simulink model "QuadrotorSimulink"  (Simulink 9.0)
settings: Solver=ode45  StartTime=0.0  StopTime=10  RelTol=1e-3  EnableMultiTasking=on
undefined symbols (not defined in the file): Quad
settings Model: Creator=test  LastModifiedBy=Dariush
settings DataIOCC: LimitDataPoints=on  SignalLoggingSaveFormat=ModelDataLogs
settings OptimizationCC: ExpressionDepthLimit=2147483647
settings DebuggingCC: FcnCallInpInsideContextMsg=warning  StateNameClashWarn=warning  StrictBusMsg=Warning
settings GRTTargetCC: CombineOutputUpdateFcns=off  GRTInterface=on

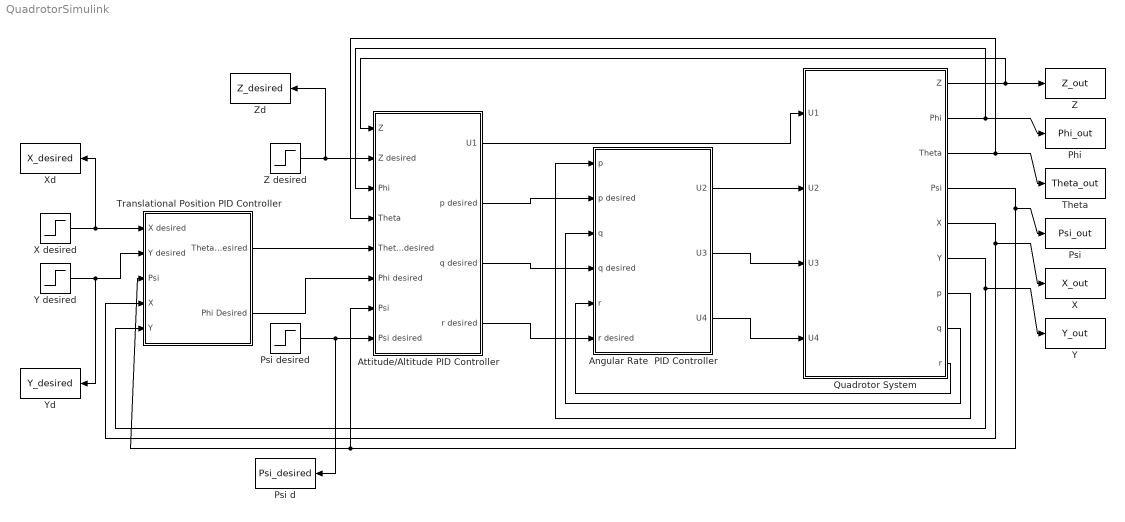
== system QuadrotorSimulink ==
  Angular Rate  PID Controller : Subsystem
  Attitude/Altitude PID Controller : Subsystem
  Phi : ToWorkspace  VariableName=Phi_out  SaveFormat=Structure  SampleTime=-1
  Psi : ToWorkspace  VariableName=Psi_out  SaveFormat=Structure  SampleTime=-1
  Psi d : ToWorkspace  VariableName=Psi_desired  SaveFormat=Structure  SampleTime=-1
  Psi desired : Step  After=0  SampleTime=0
  Quadrotor System : Subsystem
  Theta : ToWorkspace  VariableName=Theta_out  SaveFormat=Structure  SampleTime=-1
  Translational Position PID Controller : Subsystem
  X : ToWorkspace  VariableName=X_out  SaveFormat=Structure  SampleTime=-1
  X desired : Step  After=.25  SampleTime=0
  Xd : ToWorkspace  VariableName=X_desired  SaveFormat=Structure  SampleTime=-1
  Y : ToWorkspace  VariableName=Y_out  SaveFormat=Structure  SampleTime=-1
  Y desired : Step  After=0  SampleTime=0
  Yd : ToWorkspace  VariableName=Y_desired  SaveFormat=Structure  SampleTime=-1
  Z : ToWorkspace  VariableName=Z_out  SaveFormat=Structure  SampleTime=-1
  Z desired : Step  After=.5  SampleTime=0
  Zd : ToWorkspace  VariableName=Z_desired  SaveFormat=Structure  SampleTime=-1
  wires:
  Quadrotor System/2(Phi) -> Phi/1, Attitude/Altitude PID Controller/3(Phi)
  Quadrotor System/3(Theta) -> Attitude/Altitude PID Controller/4(Theta), Theta/1
  Quadrotor System/4(Psi) -> Psi/1, Translational Position PID Controller/3(Psi), Attitude/Altitude PID Controller/7(Psi)
  Quadrotor System/5(X) -> X/1, Translational Position PID Controller/4(X)
  Quadrotor System/6(Y) -> Y/1, Translational Position PID Controller/5(Y)
  Quadrotor System/1(Z) -> Attitude/Altitude PID Controller/1(Z), Z/1
  Psi desired/1 -> Attitude/Altitude PID Controller/8(Psi desired), Psi d/1
  Z desired/1 -> Attitude/Altitude PID Controller/2(Z desired), Zd/1
  X desired/1 -> Translational Position PID Controller/1(X desired), Xd/1
  Y desired/1 -> Yd/1, Translational Position PID Controller/2(Y desired)
  Attitude/Altitude PID Controller/1(U1) -> Quadrotor System/1(U1)
  Translational Position PID Controller/1(Theta Desired) -> Attitude/Altitude PID Controller/5(Theta desired)
  Translational Position PID Controller/2(Phi Desired) -> Attitude/Altitude PID Controller/6(Phi desired)
  Attitude/Altitude PID Controller/2(p desired) -> Angular Rate  PID Controller/2(p desired)
  Attitude/Altitude PID Controller/3(q desired) -> Angular Rate  PID Controller/4(q desired)
  Attitude/Altitude PID Controller/4(r desired) -> Angular Rate  PID Controller/6(r desired)
  Quadrotor System/9(r) -> Angular Rate  PID Controller/5(r)
  Quadrotor System/8(q) -> Angular Rate  PID Controller/3(q)
  Quadrotor System/7(p) -> Angular Rate  PID Controller/1(p)
  Angular Rate  PID Controller/3(U4) -> Quadrotor System/4(U4)
  Angular Rate  PID Controller/2(U3) -> Quadrotor System/3(U3)
  Angular Rate  PID Controller/1(U2) -> Quadrotor System/2(U2)

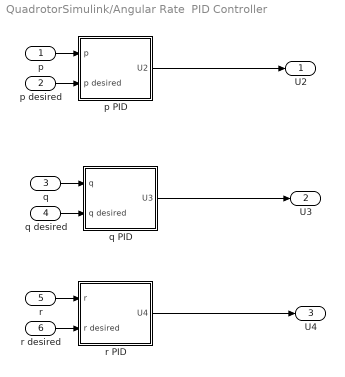
== system QuadrotorSimulink/Angular Rate  PID Controller ==
  p : Inport
  p desired : Inport  Port=2
  q : Inport  Port=3
  q desired : Inport  Port=4
  r : Inport  Port=5
  r desired : Inport  Port=6
  p PID : Subsystem
  q PID : Subsystem
  r PID : Subsystem
  U2 : Outport
  U3 : Outport  Port=2
  U4 : Outport  Port=3
  wires:
  p PID/1(U2) -> U2/1
  q PID/1(U3) -> U3/1
  r PID/1(U4) -> U4/1
  p/1 -> p PID/1(p)
  p desired/1 -> p PID/2(p desired)
  q/1 -> q PID/1(q)
  q desired/1 -> q PID/2(q desired)
  r/1 -> r PID/1(r)
  r desired/1 -> r PID/2(r desired)

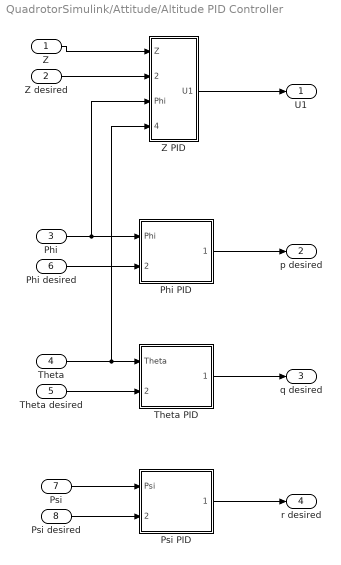
== system QuadrotorSimulink/Attitude/Altitude PID Controller ==
  Z : Inport
  Z desired : Inport  Port=2
  Phi : Inport  Port=3
  Theta : Inport  Port=4
  Theta desired : Inport  Port=5
  Phi desired : Inport  Port=6
  Psi : Inport  Port=7
  Psi desired : Inport  Port=8
  Phi PID : Subsystem
  Psi PID : Subsystem
  Theta PID : Subsystem
  Z PID : Subsystem
  U1 : Outport
  p desired : Outport  Port=2
  q desired : Outport  Port=3
  r desired : Outport  Port=4
  wires:
  Z PID/1(U1) -> U1/1
  Z desired/1 -> Z PID/2(Z desired)
  Z/1 -> Z PID/1(Z)
  Phi desired/1 -> Phi PID/2(Phi desired)
  Phi/1 -> Phi PID/1(Phi), Z PID/3(Phi)
  Psi desired/1 -> Psi PID/2(Psi desired)
  Psi/1 -> Psi PID/1(Psi)
  Theta desired/1 -> Theta PID/2(Theta desired)
  Theta/1 -> Theta PID/1(Theta), Z PID/4(Theta)
  Phi PID/1(p desired) -> p desired/1
  Psi PID/1(r desired) -> r desired/1
  Theta PID/1(q desired) -> q desired/1

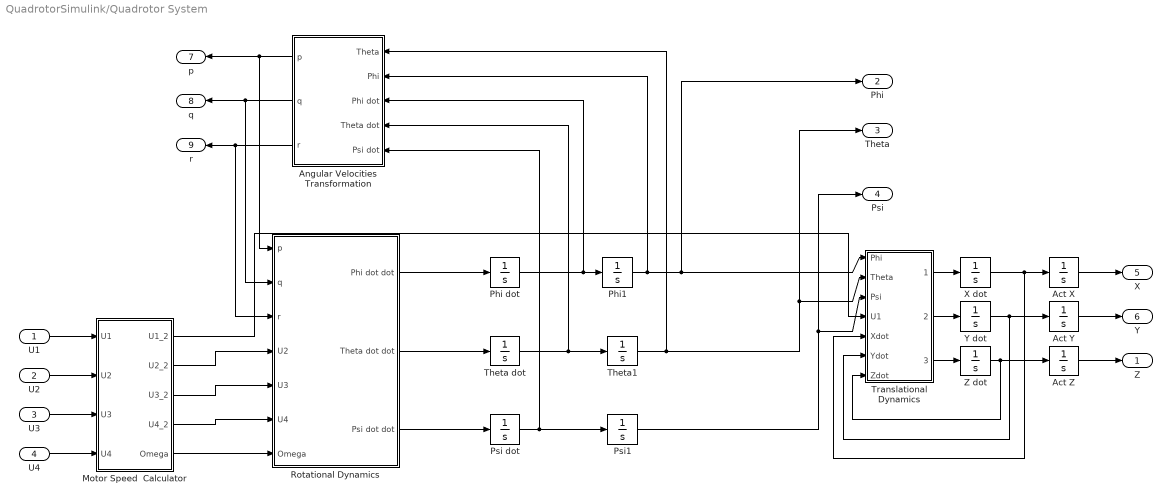
== system QuadrotorSimulink/Quadrotor System ==
  U1 : Inport
  U2 : Inport  Port=2
  U3 : Inport  Port=3
  U4 : Inport  Port=4
  Act X : Integrator
  Act Y : Integrator
  Act Z : Integrator
  Angular Velocities Transformation : Subsystem
  Motor Speed  Calculator : Subsystem
  Phi dot : Integrator
  Phi1 : Integrator  ZeroCross=off
  Psi dot : Integrator  ZeroCross=off
  Psi1 : Integrator  ZeroCross=off
  Rotational Dynamics : Subsystem
  Theta dot : Integrator  ZeroCross=off
  Theta1 : Integrator  ZeroCross=off
  Translational Dynamics : Subsystem
  X dot : Integrator
  Y dot : Integrator
  Z dot : Integrator
  Z : Outport
  Phi : Outport  Port=2
  Theta : Outport  Port=3
  Psi : Outport  Port=4
  X : Outport  Port=5
  Y : Outport  Port=6
  p : Outport  Port=7
  q : Outport  Port=8
  r : Outport  Port=9
  wires:
  Rotational Dynamics/2(Theta dot dot) -> Theta dot/1
  Motor Speed  Calculator/5(Omega) -> Rotational Dynamics/7(Omega)
  Phi1/1 -> Translational Dynamics/1(Phi), Phi/1, Angular Velocities Transformation/2(Phi)
  Theta1/1 -> Translational Dynamics/2(Theta), Theta/1, Angular Velocities Transformation/1(Theta)
  Psi1/1 -> Translational Dynamics/3(Psi), Psi/1
  Translational Dynamics/1(x dotdot) -> X dot/1
  X dot/1 -> Act X/1, Translational Dynamics/5(Xdot)
  Y dot/1 -> Act Y/1, Translational Dynamics/6(Ydot)
  Translational Dynamics/2(y dotdot) -> Y dot/1
  Z dot/1 -> Translational Dynamics/7(Zdot), Act Z/1
  Translational Dynamics/3(z dotdot) -> Z dot/1
  Act X/1 -> X/1
  Act Y/1 -> Y/1
  Act Z/1 -> Z/1
  Psi dot/1 -> Psi1/1, Angular Velocities Transformation/5(Psi dot)
  Theta dot/1 -> Theta1/1, Angular Velocities Transformation/4(Theta dot)
  Phi dot/1 -> Phi1/1, Angular Velocities Transformation/3(Phi dot)
  Rotational Dynamics/3(Psi dot dot) -> Psi dot/1
  Rotational Dynamics/1(Phi dot dot) -> Phi dot/1
  U4/1 -> Motor Speed  Calculator/4(U4)
  U2/1 -> Motor Speed  Calculator/2(U2)
  U3/1 -> Motor Speed  Calculator/3(U3)
  Motor Speed  Calculator/2(U2_2) -> Rotational Dynamics/4(U2)
  Motor Speed  Calculator/3(U3_2) -> Rotational Dynamics/5(U3)
  Motor Speed  Calculator/1(U1_2) -> Translational Dynamics/4(U1)
  Motor Speed  Calculator/4(U4_2) -> Rotational Dynamics/6(U4)
  Angular Velocities Transformation/1(p) -> Rotational Dynamics/1(p), p/1
  Angular Velocities Transformation/2(q) -> Rotational Dynamics/2(q), q/1
  Angular Velocities Transformation/3(r) -> Rotational Dynamics/3(r), r/1
  U1/1 -> Motor Speed  Calculator/1(U1)

== system QuadrotorSimulink/Translational Position PID Controller ==
  X desired : Inport
  Y desired : Inport  Port=2
  Psi : Inport  Port=3
  X : Inport  Port=4
  Y : Inport  Port=5
  Desired Position GF to BF : Subsystem
  Position GF to BF : Subsystem
  X PID : Subsystem
  Y PID : Subsystem
  Theta Desired : Outport
  Phi Desired : Outport  Port=2
  wires:
  X PID/1(Theta Desired) -> Theta Desired/1
  Y PID/1(Phi Desired) -> Phi Desired/1
  X desired/1 -> Desired Position GF to BF/1(X GF)
  Y desired/1 -> Desired Position GF to BF/2(Y GF)
  Desired Position GF to BF/1("X Bf ") -> X PID/1(X desired)
  Desired Position GF to BF/2(Y Bf) -> Y PID/1(Y desired)
  X/1 -> Position GF to BF/1(X GF)
  Y/1 -> Position GF to BF/2(Y GF)
  Position GF to BF/1("X Bf ") -> X PID/2(X)
  Position GF to BF/2(Y Bf) -> Y PID/2(Y)
  Psi/1 -> Desired Position GF to BF/3(Psi), Position GF to BF/3(Psi)

== system QuadrotorSimulink/Angular Rate  PID Controller/p PID ==
  p : Inport
  p desired : Inport  Port=2
  Derivative : Derivative
  Integrator : Integrator
  Kd : Gain  Gain=Quad.p_KD
  Ki : Gain  Gain=Quad.p_KI
  Kp : Gain  Gain=Quad.p_KP
  Psi Error : Sum  Inputs=+-
  Saturation1 : Saturate  UpperLimit=Quad.U2_max  LowerLimit=Quad.U2_min
  Sum : Sum  Inputs=+++
  U2 : Outport
  wires:
  p/1 -> Psi Error/2, Derivative/1
  p desired/1 -> Psi Error/1
  Derivative/1 -> Kd/1
  Kp/1 -> Sum/1
  Sum/1 -> U2/1
  Psi Error/1 -> Integrator/1, Kp/1
  Integrator/1 -> Ki/1
  Kd/1 -> Sum/3
  Ki/1 -> Saturation1/1
  Saturation1/1 -> Sum/2

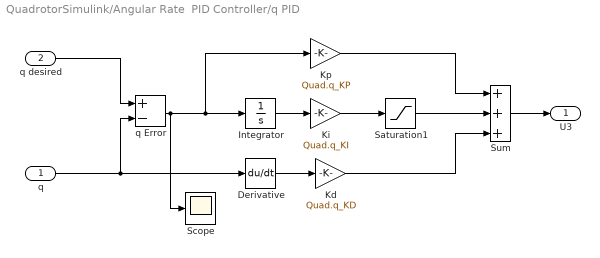
== system QuadrotorSimulink/Angular Rate  PID Controller/q PID ==
  q : Inport
  q desired : Inport  Port=2
  Derivative : Derivative
  Integrator : Integrator
  Kd : Gain  Gain=Quad.q_KD
  Ki : Gain  Gain=Quad.q_KI
  Kp : Gain  Gain=Quad.q_KP
  Saturation1 : Saturate  UpperLimit=Quad.U3_max  LowerLimit=Quad.U3_min
  Scope : Scope
  Sum : Sum  Inputs=+++
  q Error : Sum  Inputs=+-
  U3 : Outport
  wires:
  q/1 -> q Error/2, Derivative/1
  q desired/1 -> q Error/1
  Derivative/1 -> Kd/1
  Kp/1 -> Sum/1
  Sum/1 -> U3/1
  q Error/1 -> Integrator/1, Kp/1, Scope/1
  Integrator/1 -> Ki/1
  Kd/1 -> Sum/3
  Ki/1 -> Saturation1/1
  Saturation1/1 -> Sum/2

== system QuadrotorSimulink/Angular Rate  PID Controller/r PID ==
  r : Inport
  r desired : Inport  Port=2
  Derivative : Derivative
  Integrator : Integrator
  Kd : Gain  Gain=Quad.r_KD
  Ki : Gain  Gain=Quad.r_KI
  Kp : Gain  Gain=Quad.r_KP
  Psi Error : Sum  Inputs=+-
  Sum : Sum  Inputs=+++
  U4 : Outport
  wires:
  r/1 -> Psi Error/2, Derivative/1
  r desired/1 -> Psi Error/1
  Derivative/1 -> Kd/1
  Kp/1 -> Sum/1
  Sum/1 -> U4/1
  Psi Error/1 -> Integrator/1, Kp/1
  Integrator/1 -> Ki/1
  Kd/1 -> Sum/3
  Ki/1 -> Sum/2

== system QuadrotorSimulink/Attitude/Altitude PID Controller/Phi PID ==
  Phi : Inport
  Phi desired : Inport  Port=2
  Derivative : Derivative
  Integrator : Integrator
  Kd : Gain  Gain=Quad.phi_KD
  Ki : Gain  Gain=Quad.phi_KI
  Kp : Gain  Gain=Quad.phi_KP
  Psi Error : Sum  Inputs=+-
  Sum : Sum  Inputs=+++
  p desired : Outport
  wires:
  Phi/1 -> Psi Error/2, Derivative/1
  Phi desired/1 -> Psi Error/1
  Derivative/1 -> Kd/1
  Kp/1 -> Sum/1
  Sum/1 -> p desired/1
  Psi Error/1 -> Integrator/1, Kp/1
  Integrator/1 -> Ki/1
  Kd/1 -> Sum/3
  Ki/1 -> Sum/2

== system QuadrotorSimulink/Attitude/Altitude PID Controller/Psi PID ==
  Psi : Inport
  Psi desired : Inport  Port=2
  Derivative : Derivative
  Integrator : Integrator
  Kd : Gain  Gain=Quad.psi_KD
  Ki : Gain  Gain=Quad.psi_KI
  Kp : Gain  Gain=Quad.psi_KP
  Psi Error : Sum  Inputs=+-
  Sum : Sum  Inputs=+++
  r desired : Outport
  wires:
  Psi/1 -> Psi Error/2, Derivative/1
  Psi desired/1 -> Psi Error/1
  Derivative/1 -> Kd/1
  Kp/1 -> Sum/1
  Sum/1 -> r desired/1
  Psi Error/1 -> Integrator/1, Kp/1
  Integrator/1 -> Ki/1
  Kd/1 -> Sum/3
  Ki/1 -> Sum/2

== system QuadrotorSimulink/Attitude/Altitude PID Controller/Theta PID ==
  Theta : Inport
  Theta desired : Inport  Port=2
  Derivative : Derivative
  Integrator : Integrator
  Kd : Gain  Gain=Quad.theta_KD
  Ki : Gain  Gain=Quad.theta_KI
  Kp : Gain  Gain=Quad.theta_KP
  Scope : Scope
  Sum : Sum  Inputs=+++
  Theta Error : Sum  Inputs=+-
  q desired : Outport
  wires:
  Theta/1 -> Theta Error/2, Derivative/1
  Theta desired/1 -> Theta Error/1
  Derivative/1 -> Kd/1
  Kp/1 -> Sum/1
  Sum/1 -> q desired/1
  Theta Error/1 -> Integrator/1, Kp/1, Scope/1
  Integrator/1 -> Ki/1
  Kd/1 -> Sum/3
  Ki/1 -> Sum/2

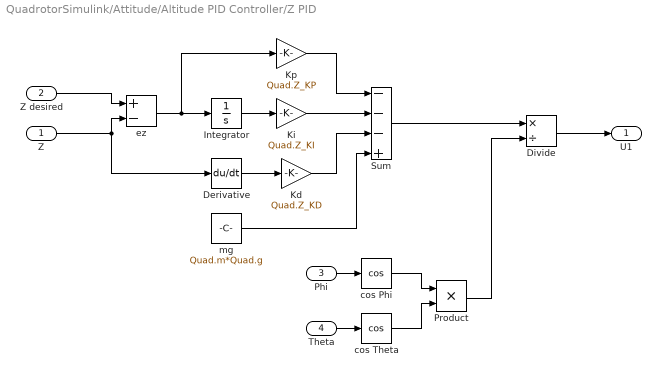
== system QuadrotorSimulink/Attitude/Altitude PID Controller/Z PID ==
  Z : Inport
  Z desired : Inport  Port=2
  Phi : Inport  Port=3
  Theta : Inport  Port=4
  Derivative : Derivative
  Divide : Product  Inputs=*/
  Integrator : Integrator
  Kd : Gain  Gain=Quad.Z_KD
  Ki : Gain  Gain=Quad.Z_KI
  Kp : Gain  Gain=Quad.Z_KP
  Product : Product  RndMeth=Zero
  Sum : Sum  Inputs=---+
  cos Phi : Trigonometry  Operator=cos
  cos Theta : Trigonometry  Operator=cos
  ez : Sum  Inputs=+-
  mg : Constant  Value=Quad.m*Quad.g
  U1 : Outport
  wires:
  Z desired/1 -> ez/1
  cos Phi/1 -> Product/1
  cos Theta/1 -> Product/2
  Product/1 -> Divide/2
  Phi/1 -> cos Phi/1
  Theta/1 -> cos Theta/1
  Z/1 -> ez/2, Derivative/1
  Derivative/1 -> Kd/1
  Kp/1 -> Sum/1
  Integrator/1 -> Ki/1
  ez/1 -> Integrator/1, Kp/1
  Sum/1 -> Divide/1
  Divide/1 -> U1/1
  mg/1 -> Sum/4
  Kd/1 -> Sum/3
  Ki/1 -> Sum/2

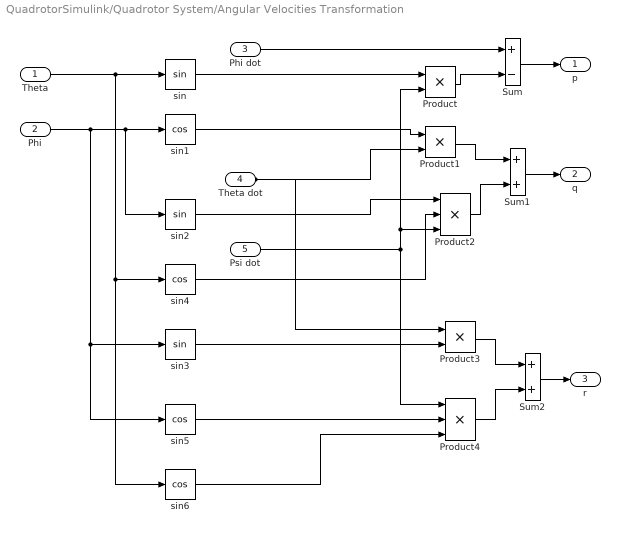
== system QuadrotorSimulink/Quadrotor System/Angular Velocities Transformation ==
  Theta : Inport
  Phi : Inport  Port=2
  Phi dot : Inport  Port=3
  Theta dot : Inport  Port=4
  Psi dot : Inport  Port=5
  Product : Product  RndMeth=Zero
  Product1 : Product  RndMeth=Zero
  Product2 : Product  Inputs=3  RndMeth=Zero
  Product3 : Product  RndMeth=Zero
  Product4 : Product  Inputs=3  RndMeth=Zero
  Sum : Sum  Inputs=+-
  Sum1 : Sum
  Sum2 : Sum
  sin : Trigonometry
  sin{1,4..6} (4 alike) : Trigonometry  Operator=cos
  sin2 : Trigonometry
  sin3 : Trigonometry
  p : Outport
  q : Outport  Port=2
  r : Outport  Port=3
  wires:
  Phi dot/1 -> Sum/1
  Theta/1 -> sin4/1, sin6/1, sin/1
  sin/1 -> Product/1
  Psi dot/1 -> Product/2, Product2/3, Product4/1
  Product/1 -> Sum/2
  Sum/1 -> p/1
  Phi/1 -> sin1/1, sin2/1, sin3/1, sin5/1
  sin1/1 -> Product1/1
  Theta dot/1 -> Product1/2, Product3/1
  Product1/1 -> Sum1/1
  sin2/1 -> Product2/1
  sin4/1 -> Product2/2
  Product2/1 -> Sum1/2
  Sum1/1 -> q/1
  sin3/1 -> Product3/2
  sin5/1 -> Product4/2
  sin6/1 -> Product4/3
  Product3/1 -> Sum2/1
  Product4/1 -> Sum2/2
  Sum2/1 -> r/1

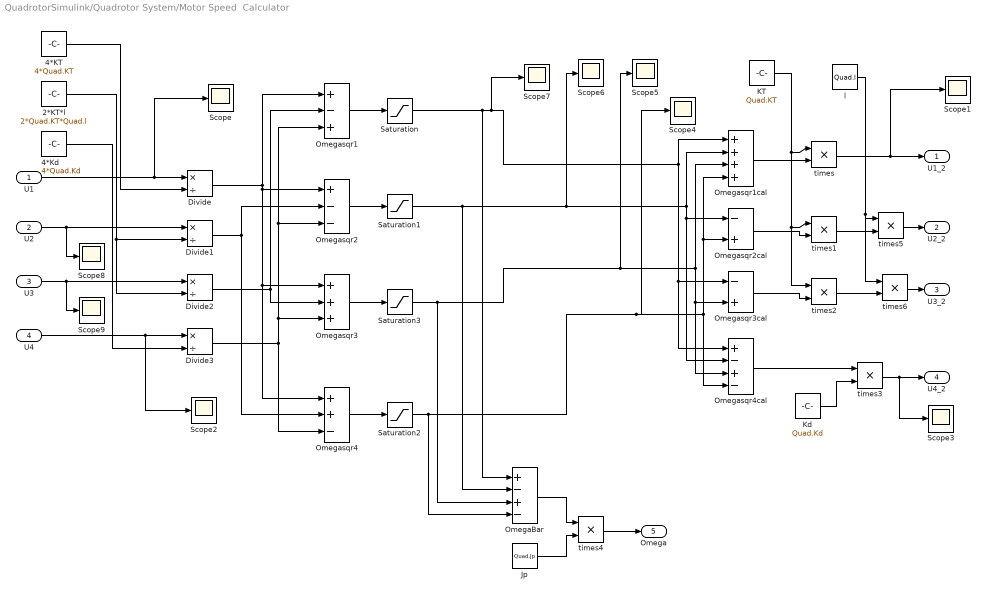
== system QuadrotorSimulink/Quadrotor System/Motor Speed  Calculator ==
  U1 : Inport
  U2 : Inport  Port=2
  U3 : Inport  Port=3
  U4 : Inport  Port=4
  2*KT*l : Constant  Value=2*Quad.KT*Quad.l
  4*KT : Constant  Value=4*Quad.KT
  4*Kd : Constant  Value=4*Quad.Kd
  Divide{,1..3} (4 alike) : Product  Inputs=*/
  Jp : Constant  Value=Quad.Jp
  KT : Constant  Value=Quad.KT
  Kd : Constant  Value=Quad.Kd
  OmegaBar : Sum  Inputs=+-+-
  Omegasqr1 : Sum  Inputs=+-+
  Omegasqr1cal : Sum  Inputs=++++
  Omegasqr2 : Sum  Inputs=+--
  Omegasqr2cal : Sum  Inputs=-+
  Omegasqr3 : Sum  Inputs=+++
  Omegasqr3cal : Sum  Inputs=-+
  Omegasqr4 : Sum  Inputs=++-
  Omegasqr4cal : Sum  Inputs=+-+-
  Saturation{,1..3} (4 alike) : Saturate  UpperLimit=Quad.max_motor_speed^2  LowerLimit=Quad.min_motor_speed^2  ZeroCross=off
  Scope{,1..9} (10 alike) : Scope
  l : Constant  Value=Quad.l
  times{,1..6} (7 alike) : Product  Inputs=**
  U1_2 : Outport
  U2_2 : Outport  Port=2
  U3_2 : Outport  Port=3
  U4_2 : Outport  Port=4
  Omega : Outport  Port=5
  wires:
  U1/1 -> Divide/1, Scope/1
  4*KT/1 -> Divide/2
  U2/1 -> Divide1/1, Scope8/1
  2*KT*l/1 -> Divide1/2, Divide2/2
  U3/1 -> Divide2/1, Scope9/1
  U4/1 -> Divide3/1, Scope2/1
  4*Kd/1 -> Divide3/2
  Divide/1 -> Omegasqr1/1, Omegasqr2/1, Omegasqr3/1, Omegasqr4/1
  Divide2/1 -> Omegasqr1/2, Omegasqr3/2
  Divide3/1 -> Omegasqr1/3, Omegasqr2/3, Omegasqr3/3, Omegasqr4/3
  Divide1/1 -> Omegasqr2/2, Omegasqr4/2
  OmegaBar/1 -> times4/1
  times4/1 -> Omega/1
  KT/1 -> times/1, times1/1, times2/1
  Omegasqr1cal/1 -> times/2
  Omegasqr2cal/1 -> times1/2
  Omegasqr3cal/1 -> times2/2
  Omegasqr4cal/1 -> times3/1
  Kd/1 -> times3/2
  times/1 -> U1_2/1, Scope1/1
  times3/1 -> U4_2/1, Scope3/1
  Jp/1 -> times4/2
  times5/1 -> U2_2/1
  times6/1 -> U3_2/1
  l/1 -> times5/1, times6/1
  times1/1 -> times5/2
  times2/1 -> times6/2
  Saturation/1 -> OmegaBar/1, Omegasqr1cal/1, Omegasqr3cal/1, Omegasqr4cal/1, Scope7/1
  Saturation2/1 -> OmegaBar/4, Omegasqr1cal/4, Omegasqr2cal/2, Omegasqr4cal/4, Scope4/1
  Saturation3/1 -> OmegaBar/3, Omegasqr1cal/3, Omegasqr3cal/2, Omegasqr4cal/3, Scope5/1
  Saturation1/1 -> OmegaBar/2, Omegasqr1cal/2, Omegasqr2cal/1, Omegasqr4cal/2, Scope6/1
  Omegasqr1/1 -> Saturation/1
  Omegasqr2/1 -> Saturation1/1
  Omegasqr3/1 -> Saturation3/1
  Omegasqr4/1 -> Saturation2/1

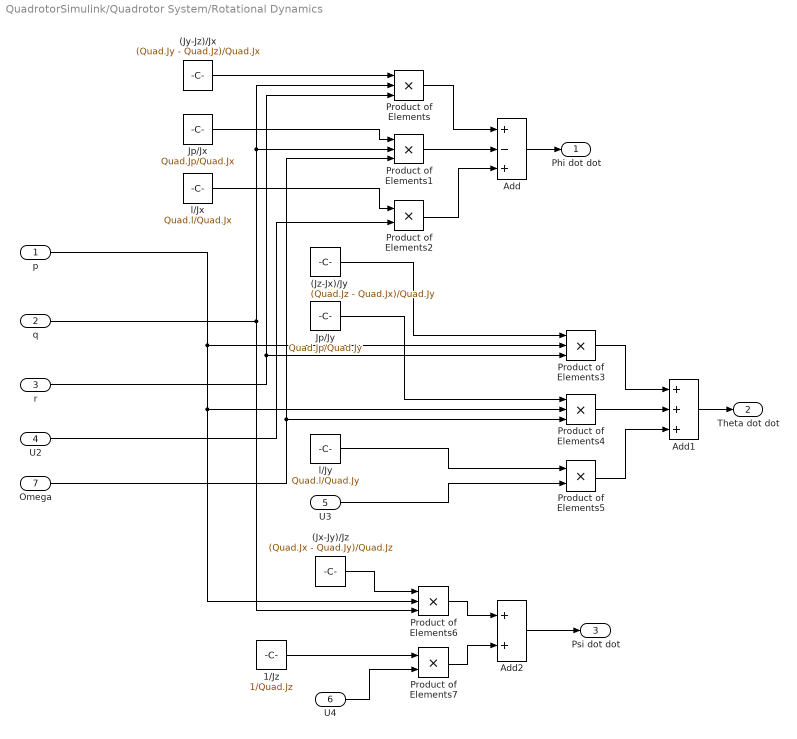
== system QuadrotorSimulink/Quadrotor System/Rotational Dynamics ==
  p : Inport
  q : Inport  Port=2
  r : Inport  Port=3
  U2 : Inport  Port=4
  U3 : Inport  Port=5
  U4 : Inport  Port=6
  Omega : Inport  Port=7
  (Jx-Jy)/Jz : Constant  Value=(Quad.Jx - Quad.Jy)/Quad.Jz
  (Jy-Jz)/Jx : Constant  Value=(Quad.Jy - Quad.Jz)/Quad.Jx
  (Jz-Jx)/Jy : Constant  Value=(Quad.Jz - Quad.Jx)/Quad.Jy
  1/Jz : Constant  Value=1/Quad.Jz
  Add : Sum  Inputs=+-+
  Add1 : Sum  Inputs=+++
  Add2 : Sum
  Jp/Jx : Constant  Value=Quad.Jp/Quad.Jx
  Jp/Jy : Constant  Value=Quad.Jp/Quad.Jy
  Product of Elements{,1,3..4,6} (5 alike) : Product  Inputs=3
  Product of Elements2 : Product
  Product of Elements5 : Product
  Product of Elements7 : Product
  l/Jx : Constant  Value=Quad.l/Quad.Jx
  l/Jy : Constant  Value=Quad.l/Quad.Jy
  Phi dot dot : Outport
  Theta dot dot : Outport  Port=2
  Psi dot dot : Outport  Port=3
  wires:
  Product of Elements/1 -> Add/1
  Product of Elements1/1 -> Add/2
  Product of Elements2/1 -> Add/3
  Add/1 -> Phi dot dot/1
  (Jy-Jz)/Jx/1 -> Product of Elements/1
  q/1 -> Product of Elements/2, Product of Elements1/2, Product of Elements6/3
  r/1 -> Product of Elements/3, Product of Elements3/3
  Jp/Jx/1 -> Product of Elements1/1
  l/Jx/1 -> Product of Elements2/1
  U2/1 -> Product of Elements2/2
  Omega/1 -> Product of Elements1/3, Product of Elements4/3
  Product of Elements3/1 -> Add1/1
  Product of Elements4/1 -> Add1/2
  Product of Elements5/1 -> Add1/3
  Add1/1 -> Theta dot dot/1
  (Jz-Jx)/Jy/1 -> Product of Elements3/1
  Jp/Jy/1 -> Product of Elements4/1
  l/Jy/1 -> Product of Elements5/1
  U3/1 -> Product of Elements5/2
  p/1 -> Product of Elements3/2, Product of Elements4/2, Product of Elements6/2
  Product of Elements7/1 -> Add2/2
  Add2/1 -> Psi dot dot/1
  U4/1 -> Product of Elements7/2
  1/Jz/1 -> Product of Elements7/1
  (Jx-Jy)/Jz/1 -> Product of Elements6/1
  Product of Elements6/1 -> Add2/1

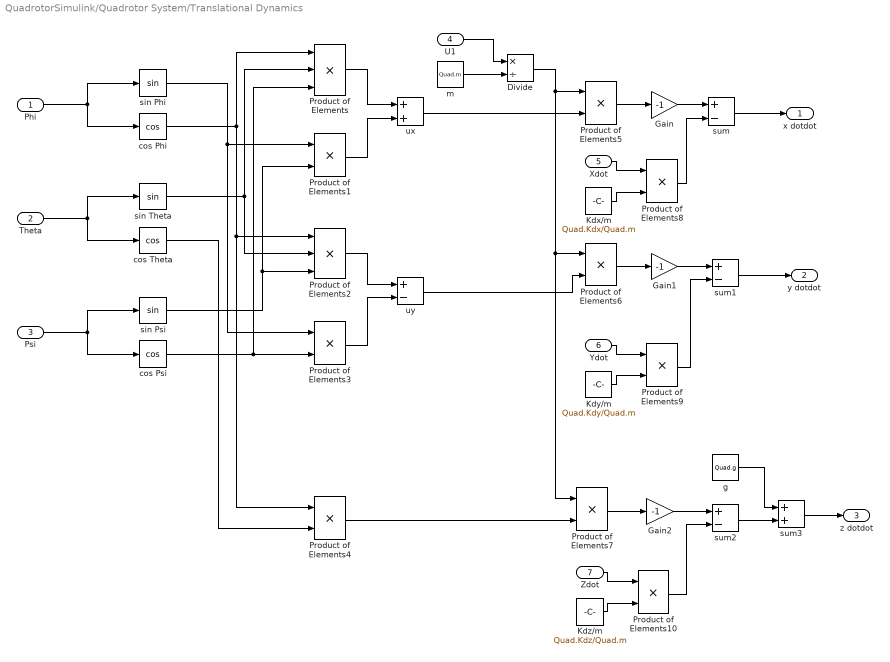
== system QuadrotorSimulink/Quadrotor System/Translational Dynamics ==
  Phi : Inport
  Theta : Inport  Port=2
  Psi : Inport  Port=3
  U1 : Inport  Port=4
  Xdot : Inport  Port=5
  Ydot : Inport  Port=6
  Zdot : Inport  Port=7
  Divide : Product  Inputs=*/
  Gain : Gain  Gain=-1
  Gain1 : Gain  Gain=-1
  Gain2 : Gain  Gain=-1
  Kdx/m : Constant  Value=Quad.Kdx/Quad.m
  Kdy/m : Constant  Value=Quad.Kdy/Quad.m
  Kdz/m : Constant  Value=Quad.Kdz/Quad.m
  Product of Elements : Product  Inputs=3
  Product of Elements{1,3..10} (9 alike) : Product
  Product of Elements2 : Product  Inputs=3
  cos Phi : Trigonometry  Operator=cos
  cos Psi : Trigonometry  Operator=cos
  cos Theta : Trigonometry  Operator=cos
  g : Constant  Value=Quad.g
  m : Constant  Value=Quad.m
  sin Phi : Trigonometry
  sin Psi : Trigonometry
  sin Theta : Trigonometry
  sum : Sum  Inputs=+-
  sum1 : Sum  Inputs=+-
  sum2 : Sum  Inputs=+-
  sum3 : Sum
  ux : Sum
  uy : Sum  Inputs=+-
  x dotdot : Outport
  y dotdot : Outport  Port=2
  z dotdot : Outport  Port=3
  wires:
  Phi/1 -> sin Phi/1, cos Phi/1
  Theta/1 -> sin Theta/1, cos Theta/1
  Psi/1 -> sin Psi/1, cos Psi/1
  sin Theta/1 -> Product of Elements/2, Product of Elements2/2
  cos Psi/1 -> Product of Elements/3, Product of Elements3/2
  cos Phi/1 -> Product of Elements/1, Product of Elements2/1, Product of Elements4/1
  sin Phi/1 -> Product of Elements1/1, Product of Elements3/1
  sin Psi/1 -> Product of Elements1/2, Product of Elements2/3
  Product of Elements/1 -> ux/1
  Product of Elements1/1 -> ux/2
  ux/1 -> Product of Elements5/2
  Product of Elements2/1 -> uy/1
  Product of Elements3/1 -> uy/2
  uy/1 -> Product of Elements6/2
  cos Theta/1 -> Product of Elements4/2
  Product of Elements4/1 -> Product of Elements7/2
  U1/1 -> Divide/1
  m/1 -> Divide/2
  Divide/1 -> Product of Elements5/1, Product of Elements6/1, Product of Elements7/1
  sum3/1 -> z dotdot/1
  Product of Elements5/1 -> Gain/1
  Product of Elements6/1 -> Gain1/1
  Xdot/1 -> Product of Elements8/1
  Kdx/m/1 -> Product of Elements8/2
  Gain/1 -> sum/1
  Product of Elements8/1 -> sum/2
  sum/1 -> x dotdot/1
  Ydot/1 -> Product of Elements9/1
  Kdy/m/1 -> Product of Elements9/2
  Gain1/1 -> sum1/1
  Product of Elements9/1 -> sum1/2
  sum1/1 -> y dotdot/1
  Zdot/1 -> Product of Elements10/1
  Kdz/m/1 -> Product of Elements10/2
  Product of Elements7/1 -> Gain2/1
  g/1 -> sum3/1
  sum2/1 -> sum3/2
  Product of Elements10/1 -> sum2/2
  Gain2/1 -> sum2/1

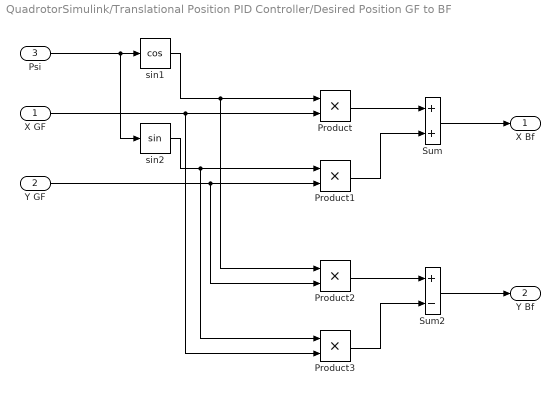
== system QuadrotorSimulink/Translational Position PID Controller/Desired Position GF to BF ==
  X GF : Inport
  Y GF : Inport  Port=2
  Psi : Inport  Port=3
  Product{,1..3} (4 alike) : Product  RndMeth=Zero
  Sum : Sum
  Sum2 : Sum  Inputs=+-
  sin1 : Trigonometry  Operator=cos
  sin2 : Trigonometry
  "X Bf " : Outport
  Y Bf : Outport  Port=2
  wires:
  Psi/1 -> sin1/1, sin2/1
  sin1/1 -> Product/1, Product2/1
  X GF/1 -> Product/2, Product3/2
  Product/1 -> Sum/1
  sin2/1 -> Product1/1, Product3/1
  Y GF/1 -> Product1/2, Product2/2
  Product1/1 -> Sum/2
  Sum/1 -> "X Bf "/1
  Product2/1 -> Sum2/1
  Product3/1 -> Sum2/2
  Sum2/1 -> Y Bf/1

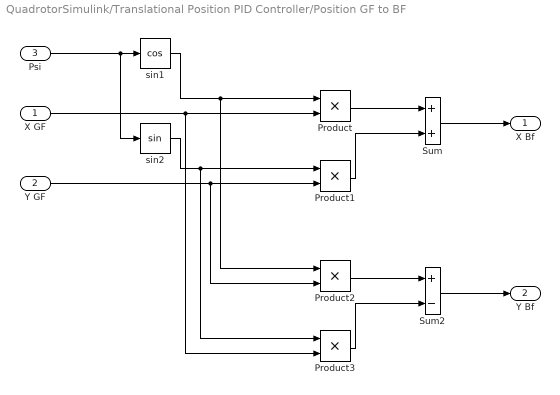
== system QuadrotorSimulink/Translational Position PID Controller/Position GF to BF ==
  X GF : Inport
  Y GF : Inport  Port=2
  Psi : Inport  Port=3
  Product{,1..3} (4 alike) : Product  RndMeth=Zero
  Sum : Sum
  Sum2 : Sum  Inputs=+-
  sin1 : Trigonometry  Operator=cos
  sin2 : Trigonometry
  "X Bf " : Outport
  Y Bf : Outport  Port=2
  wires:
  Psi/1 -> sin1/1, sin2/1
  sin1/1 -> Product/1, Product2/1
  X GF/1 -> Product/2, Product3/2
  Product/1 -> Sum/1
  sin2/1 -> Product1/1, Product3/1
  Y GF/1 -> Product1/2, Product2/2
  Product1/1 -> Sum/2
  Sum/1 -> "X Bf "/1
  Product2/1 -> Sum2/1
  Product3/1 -> Sum2/2
  Sum2/1 -> Y Bf/1

== system QuadrotorSimulink/Translational Position PID Controller/X PID ==
  X desired : Inport
  X : Inport  Port=2
  Derivative : Derivative
  Integrator : Integrator
  Kd : Gain  Gain=Quad.X_KD
  Ki : Gain  Gain=Quad.X_KI
  Kp : Gain  Gain=Quad.X_KP
  Saturation1 : Saturate  UpperLimit=Quad.theta_max  LowerLimit=-Quad.theta_max
  Saturation2 : Saturate  UpperLimit=Quad.theta_max  LowerLimit=-Quad.theta_max
  Sum : Sum  Inputs=---
  X Error : Sum  Inputs=+-
  Theta Desired : Outport
  wires:
  X/1 -> X Error/2, Derivative/1
  X desired/1 -> X Error/1
  Derivative/1 -> Kd/1
  Kp/1 -> Sum/1
  Sum/1 -> Saturation2/1
  X Error/1 -> Integrator/1, Kp/1
  Integrator/1 -> Ki/1
  Kd/1 -> Sum/3
  Saturation2/1 -> Theta Desired/1
  Ki/1 -> Saturation1/1
  Saturation1/1 -> Sum/2

== system QuadrotorSimulink/Translational Position PID Controller/Y PID ==
  Y desired : Inport
  Y : Inport  Port=2
  Derivative : Derivative
  Integrator : Integrator
  Kd : Gain  Gain=Quad.Y_KD
  Ki : Gain  Gain=Quad.Y_KI
  Kp : Gain  Gain=Quad.Y_KP
  Saturation1 : Saturate  UpperLimit=Quad.phi_max  LowerLimit=-Quad.phi_max
  Saturation2 : Saturate  UpperLimit=Quad.phi_max  LowerLimit=-Quad.phi_max
  Sum : Sum  Inputs=+++
  Y Error : Sum  Inputs=+-
  Phi Desired : Outport
  wires:
  Y/1 -> Y Error/2, Derivative/1
  Y desired/1 -> Y Error/1
  Derivative/1 -> Kd/1
  Kp/1 -> Sum/1
  Sum/1 -> Saturation2/1
  Y Error/1 -> Integrator/1, Kp/1
  Integrator/1 -> Ki/1
  Kd/1 -> Sum/3
  Ki/1 -> Saturation1/1
  Saturation1/1 -> Sum/2
  Saturation2/1 -> Phi Desired/1
